simulink model "threephaseinverter_1"  (Simulink 6.0)
settings: Solver=ode23tb  StartTime=0.0  StopTime=0.06  RelTol=1e-3
libraries: powerlib x7, powerlib_extras x1, simulink x1
settings Model: LastModifiedBy=Administrator

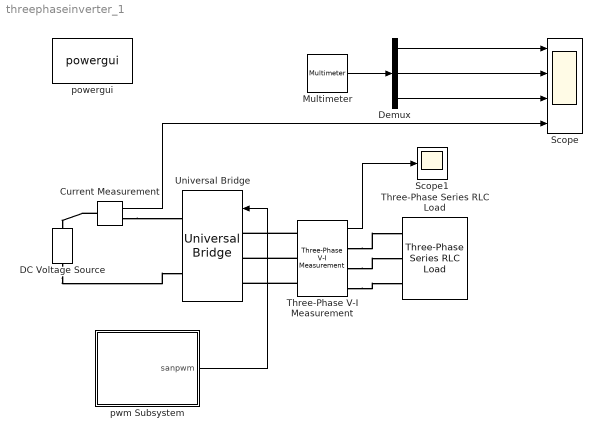
== system threephaseinverter_1 ==
  Current Measurement : powerlib/Measurements/Current Measurement  PhasorSimulation=off  OutputType=Complex  PSBequivalent=0
  DC Voltage Source : powerlib/Electrical Sources/DC Voltage Source  Orientation=up  Amplitude=300  Measurements=None
  Demux : Demux  Outputs=3
  Multimeter : powerlib/Measurements/Multimeter  PhasorSimulation=off  OutputType=Complex  sel=[1 4 5]  L=6  Gain=[1 1 1]  yselected={'Uag: Three-Phase Series RLC Load','Iag: Three-Phase Series RLC Load','Ibg: Three-Phase Series RLC Load'};  PSBOutputType=1  PSBequivalent=0  AxesSetting=[0,0.1,-100,100]  Display=0  SavedBlockNames=-11
  Scope : Scope  NumInputPorts=4
      settings: TimeRange=0.06  YMin=-200~-5~-5~0  YMax=200~5~5~4  SaveName=t_Data
  Scope1 : Scope
      settings: DataFormat=Array
  Three-Phase Series RLC Load : powerlib/Elements/Three-Phase Series RLC Load  PhysicalDomain=powersysdomain  SubClassName=unknown  LeftPortType=p1  RightPortType=p1  LConnTagsString=A|B|C  Configuration=Y (grounded)  NominalVoltage=208  NominalFrequency=50  ActivePower=1e3  InductivePower=500  CapacitivePower=0  Measurements=Branch voltages and currents
  Three-Phase V-I Measurement : powerlib/Measurements/Three-Phase V-I Measurement  VoltageMeasurement=phase-to-ground  SetLabelV=on  LabelV=Vabc  Vpu=on  Vbase=500e3  CurrentMeasurement=yes  SetLabelI=off  LabelI=Iabc  Ipu=off  Pbase=100e6  OutputType=Complex  PhasorSimulation=off  PSBequivalent=0
  Universal Bridge : powerlib/Power Electronics/Universal Bridge  Orientation=left  Arms=3  SnubberResistance=1e5  SnubberCapacitance=inf  Device=MOSFET / Diodes  Ron=1e-3  Lon=0  ForwardVoltages="[  0  0  ]"  ForwardVoltage=0  GTOparameters=[ 10e-6 , 20e-6 ]  IGBTparameters=[ 1e-6 , 2e-6 ]  Measurements=None
  powergui : powerlib/powergui  Priority=2  Frange=[0:2:500]  Ylog=off  Xlog=on  save=off  variable=ZData  structure=t_Data  ZoomFFT=on  StartTime=0.0  cycles=2  DisplayStyle=1  fundamental=50  FreqAxis=on  MaxFrequency=1000  frequencyindice=1  frequencyindicesteady=1  RmsSteady=1  display=off  Ts=5e-7  methode=off  frequency=50  echomessages=off
  pwm Subsystem : Subsystem  mask{Ts=5e-7}
      mask prompts: Ts "sampling time(s)"
  wires:
  pwm Subsystem/1(sanpwm) -> Universal Bridge/1
  Multimeter/1 -> Demux/1
  Demux/1 -> Scope/1
  Demux/2 -> Scope/2
  Demux/3 -> Scope/3
  Current Measurement/1 -> Scope/4
  Three-Phase V-I Measurement/1 -> Scope1/1
  connections:
  Current Measurement/LConn1 -- DC Voltage Source/RConn1
  Current Measurement/RConn1 -- Universal Bridge/RConn1
  DC Voltage Source/LConn1 -- Universal Bridge/RConn2
  Three-Phase V-I Measurement/LConn1 -- Universal Bridge/LConn1
  Three-Phase V-I Measurement/LConn2 -- Universal Bridge/LConn2
  Three-Phase V-I Measurement/LConn3 -- Universal Bridge/LConn3
  Three-Phase V-I Measurement/RConn3 -- Three-Phase Series RLC Load/LConn3
  Three-Phase V-I Measurement/RConn2 -- Three-Phase Series RLC Load/LConn2
  Three-Phase V-I Measurement/RConn1 -- Three-Phase Series RLC Load/LConn1

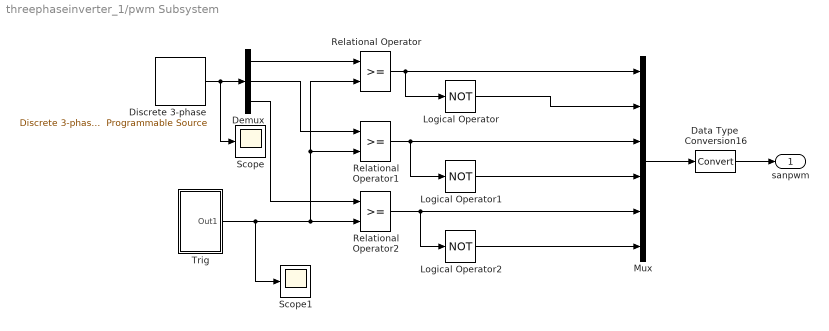
== system threephaseinverter_1/pwm Subsystem ==
  Data Type  Conversion16 : DataTypeConversion  OutDataTypeMode=double  SaturateOnIntegerOverflow=on  RndMeth=Zero
  Demux : Demux  Outputs=3
  "Discrete 3-phase " : powerlib_extras/Discrete  Control Blocks/Discrete 3-phase  Programmable Source  Par_Vps=[0.8 0 50]  VariationEntity=None  VariationType=Step  VariationStep=-0.5  VariationRate=10  VariationMag=0.3  VariationFreq=2  Par_Timing_Variation=[0.1 1.2]  SinglePhase=on  Yampli=[1 0.8 1.2 1.0]  Xtime=[0 0.1 0.15 0.2]  HarmonicGeneration=off  Par_HarmoA=[3 0.2 -25 0]  Par_HarmoB=[2 0.15 35 2]  Par_Timing_Harmo="[0.05  3]"  Ts=Ts
  Logical Operator : Logic  Operator=NOT  Inputs=1  AllPortsSameDT=off  OutDataTypeMode=Boolean
  Logical Operator1 : Logic  Operator=NOT  Inputs=1  AllPortsSameDT=off  OutDataTypeMode=Boolean
  Logical Operator2 : Logic  Operator=NOT  Inputs=1  AllPortsSameDT=off  OutDataTypeMode=Boolean
  Mux : Mux  Inputs=6
  Relational Operator : RelationalOperator  LogicOutDataTypeMode=Boolean
  Relational Operator1 : RelationalOperator  LogicOutDataTypeMode=Boolean
  Relational Operator2 : RelationalOperator  LogicOutDataTypeMode=Boolean
  Scope : Scope
      settings: DataFormat=Array
  Scope1 : Scope
      settings: SaveName=ScopeData2  DataFormat=Array
  Trig : Subsystem  mask{Fc=1500}
      mask prompts: Fc "Carrier Frequency(Hz)"
  sanpwm : Outport
  wires:
  "Discrete 3-phase "/1 -> Demux/1, Scope/1
  Demux/3 -> Relational Operator2/1
  Demux/1 -> Relational Operator/1
  Demux/2 -> Relational Operator1/1
  Trig/1(Out1) -> Relational Operator2/2, Relational Operator/2, Relational Operator1/2, Scope1/1
  Relational Operator/1 -> Logical Operator/1, Mux/1
  Relational Operator1/1 -> Logical Operator1/1, Mux/3
  Relational Operator2/1 -> Logical Operator2/1, Mux/5
  Mux/1 -> Data Type  Conversion16/1
  Data Type  Conversion16/1 -> sanpwm/1
  Logical Operator/1 -> Mux/2
  Logical Operator1/1 -> Mux/4
  Logical Operator2/1 -> Mux/6

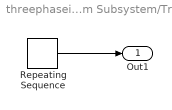
== system threephaseinverter_1/pwm Subsystem/Trig ==
  Repeating Sequence : simulink/Sources/Repeating Sequence  rep_seq_t=[0 1/Fc/4 3/Fc/4 1/Fc]  rep_seq_y=[0 1 -1 0]
  Out1 : Outport
  wires:
  Repeating Sequence/1 -> Out1/1
